simulink model "mavlink"  (R2024b)
settings: Solver=VariableStepAuto  StartTime=0.0  StopTime=10.0  RelTol=1e-3
settings Model: Creator=CETCA  LastModifiedBy=CETCA

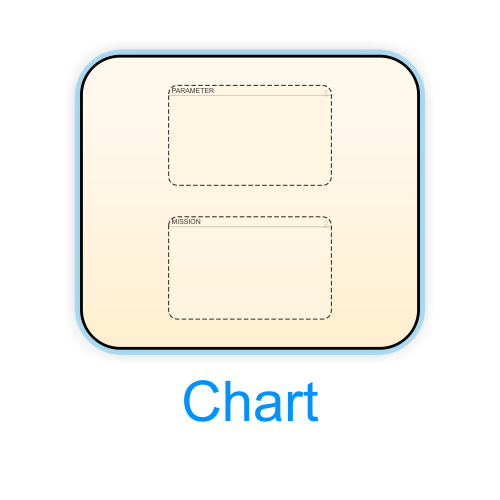
[thumbnail: Simulink's stored preview of the top-level diagram]
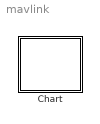
== system mavlink ==
  Chart : Stateflow chart  TreatAsAtomicUnit=on

== stateflow chart mavlink/Chart ==
  state PING [parallel]
    settings: executionOrder=2
    note: ?
  state HEARTBEAT [parallel]
    settings: executionOrder=1
  state COMMAND [parallel]
    settings: executionOrder=5
    note: ?
  state MISSION [parallel]
    settings: executionOrder=4
    state MISSION_DOWNLOAD
      note: ?
      state MISSION_COUNT
      state MISSION_REQUEST_INT
      state MISSION_ITEM_INT
      state MISSION_ACK
      (default) -> MISSION_COUNT
      MISSION_COUNT -> MISSION.MISSION_DOWNLOAD.MISSION_REQUEST_INT
      MISSION.MISSION_DOWNLOAD.MISSION_REQUEST_INT -> MISSION.MISSION_DOWNLOAD.MISSION_ITEM_INT
      MISSION.MISSION_DOWNLOAD.MISSION_ITEM_INT -> MISSION.MISSION_DOWNLOAD.MISSION_REQUEST_INT [order 1]
      MISSION.MISSION_DOWNLOAD.MISSION_ITEM_INT -> MISSION.MISSION_DOWNLOAD.MISSION_ACK [order 2]
    state MISSION_IDEL
    state MISSION_CLEAR_ALL
      note: ?
    state MISSION_SET_CURRENT
      note: ?
    state MISSION_UPLOAD
      note: ?
      state MISSION_REQUEST_INT
      state MISSION_ITEM_INT
      state MISSION_ACK
      (default) -> MISSION.MISSION_UPLOAD.MISSION_REQUEST_INT
      MISSION.MISSION_UPLOAD.MISSION_REQUEST_INT -> MISSION.MISSION_UPLOAD.MISSION_ITEM_INT
      MISSION.MISSION_UPLOAD.MISSION_ITEM_INT -> MISSION.MISSION_UPLOAD.MISSION_REQUEST_INT [order 1]
      MISSION.MISSION_UPLOAD.MISSION_ITEM_INT -> MISSION.MISSION_UPLOAD.MISSION_ACK [order 2]
    MISSION_DOWNLOAD -> MISSION_IDEL
    MISSION_IDEL -> MISSION_DOWNLOAD [order 2] : MISSION_REQUEST_LIST
    (default) -> MISSION_IDEL
    MISSION_CLEAR_ALL -> MISSION_IDEL
    MISSION_SET_CURRENT -> MISSION_IDEL
    MISSION_IDEL -> MISSION_CLEAR_ALL [order 3]
    MISSION_IDEL -> MISSION_SET_CURRENT [order 4]
    MISSION_IDEL -> MISSION_UPLOAD [order 1] : MISSION_COUNT
    MISSION_UPLOAD -> MISSION_IDEL
  state PARAMETER [parallel]
    settings: executionOrder=3
    state READ_PARAM
      % 返回PARAM_VALUE
      note: ?
    state WRITE_PARAM
      % 返回PARAM_VALUE
      note: ?
    state PARAM_IDEL
    state REAL_ALL_PARAM
      note: ?
      state PARAM_VALUE
      (default) -> PARAM_VALUE
      PARAM_VALUE -> PARAM_VALUE
    (default) -> PARAM_IDEL
    READ_PARAM -> PARAM_IDEL
    WRITE_PARAM -> PARAM_IDEL
    PARAM_IDEL -> READ_PARAM [order 2] : PARAM_RQUEST_READ
    PARAM_IDEL -> WRITE_PARAM [order 3] : PARAM_SET
    PARAM_IDEL -> REAL_ALL_PARAM [order 1] : PARAM_REQUEST_LIST
    REAL_ALL_PARAM -> REAL_ALL_PARAM : PARAM_REQUEST_LIST
